simulink model "EncoderLIDARtrial"  (R2015a)
settings: Solver=ode3  StartTime=0.0  StopTime=inf  RelTol=1e-3
settings Model: SimulationMode=external  ExtModeTrigDuration=100  Creator=Justin  LastModifiedBy=Will
settings OptimizationCC: OptimizeModelRefInitCode=on  LifeSpan=Inf
settings HardwareCC: ProdLargestAtomicInteger=Long  ProdLargestAtomicFloat=Double  ProdEndianess=LittleEndian  ProdHWDeviceType=ARM Compatible->ARM Cortex
settings RTWCC: SystemTargetFile=realtime.tlc  GenerateMakefile=off  TemplateMakefile=realtime.tmf  Description=Run on Target Hardware  RTWVerbose=off
settings ERTTargetCC: CombineOutputUpdateFcns=off  ExtMode=on  ExtModeMexArgs='169.254.0.2' 0 17725 30  ERTSrcFileBannerTemplate=realtime_code_template.cgt  ERTHdrFileBannerTemplate=realtime_code_template.cgt  ERTDataSrcFileTemplate=realtime_code_template.cgt  ERTDataHdrFileTemplate=realtime_code_template.cgt  ERTCustomFileTemplate=realtime_file_process.tlc

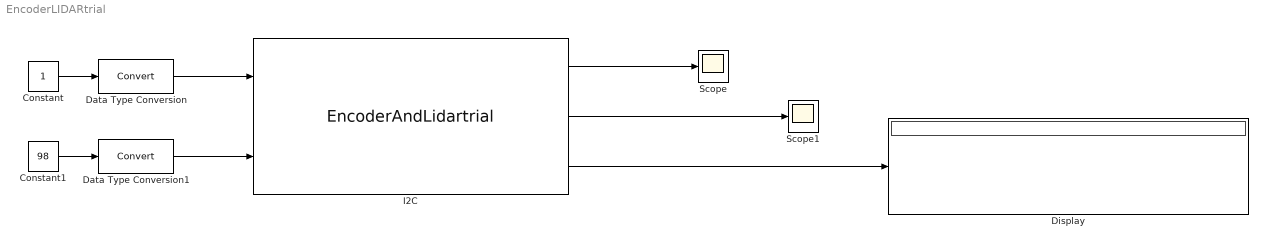
== system EncoderLIDARtrial ==
  Constant : Constant
  Constant1 : Constant  Value=98
  Data Type Conversion : DataTypeConversion
  Data Type Conversion1 : DataTypeConversion
  Display : Display
  I2C : S-Function  InitFcn=try, set_param(gcb,'FunctionName','EncoderAndLidartrial'), end  FunctionName=EncoderAndLidartrial  SFunctionModules=EncoderAndLidartrial_wrapper  mask(S-Function Builder){}
      mask init:
      | val = [[.9  0.75 0.75 1 1 .9 .9 1]',[1 1 0.75 0.75 .9 .9 1 .9]'];try , sys = get_param(gcb,'SfunBuilderFcnName');if isempty(sys), sys = get_param(gcb,'FunctionName'); end,catch, sys = get_param(gcb,'FunctionName'); end
      settings: CopyFcn=set_param(gcbh,'LinkStatus','none')  PreSaveFcn=try, set_param(gcb,'FunctionName','EncoderAndLidartrial'), end  OpenFcn=sfunctionwizard(gcbh)
      mask Display: plot(val(:,1),val(:,2)),disp(sys), port_label('input',1,'Bus'), port_label('input',2,'DeviceAddr'), port_label('output',1,'Register_Value1'), port_label('output',2,'Register_Value2'), port_label('output',3,'RegValue')
  Scope : Scope
      settings: YMin=0  YMax=110
  Scope1 : Scope
      settings: YMin=4.08022e+09  YMax=4.50972e+09
  wires:
  I2C/1 -> Scope/1
  I2C/2 -> Scope1/1
  Data Type Conversion1/1 -> I2C/2
  Constant1/1 -> Data Type Conversion1/1
  Constant/1 -> Data Type Conversion/1
  Data Type Conversion/1 -> I2C/1
  I2C/3 -> Display/1
